simulink model "Starfighter_6DoF_runsim_waypoint"  (R2013b)
settings: Solver=ode4  StartTime=0.0  StopTime=1  FixedStep=.01  MaxStep=.004  RelTol=1e-5
values from neighbouring files (symbols this model uses):
  a = 967.78    [LocusTrans.m]    (also in runsim_Starfighter_6DoF_Waypoint.m)
  ac = [0 0 0]    [LocusTrans.m]    (also in runsim_Starfighter_6DoF_Waypoint.m)
  b = 21.9    [LocusTrans.m]    (also in runsim_Starfighter_6DoF_Waypoint.m)
  cbar = 9.6    [LocusTrans.m]    (also in runsim_Starfighter_6DoF_Waypoint.m)
  cda = 0.384    [LocusTrans.m]    (also in runsim_Starfighter_6DoF_Waypoint.m)
  cdde = 0    [LocusTrans.m]    (also in runsim_Starfighter_6DoF_Waypoint.m)
  cdo = 0.048    [LocusTrans.m]    (also in runsim_Starfighter_6DoF_Waypoint.m)
  cg = [0 0 0]    [LocusTrans.m]    (also in runsim_Starfighter_6DoF_Waypoint.m)
  cla = 2.005    [LocusTrans.m]    (also in runsim_Starfighter_6DoF_Waypoint.m)
  cladot = 0.82    [LocusTrans.m]    (also in runsim_Starfighter_6DoF_Waypoint.m)
  clb = -0.093    [LocusTrans.m]    (also in runsim_Starfighter_6DoF_Waypoint.m)
  clda = 0.0173    [LocusTrans.m]    (also in runsim_Starfighter_6DoF_Waypoint.m)
  clde = 0.523    [LocusTrans.m]    (also in runsim_Starfighter_6DoF_Waypoint.m)
  cldr = 0.0079    [LocusTrans.m]    (also in runsim_Starfighter_6DoF_Waypoint.m)
  clo = 0.122    [LocusTrans.m]    (also in runsim_Starfighter_6DoF_Waypoint.m)
  clp = -0.272    [LocusTrans.m]    (also in runsim_Starfighter_6DoF_Waypoint.m)
  clq = 1.9    [LocusTrans.m]    (also in runsim_Starfighter_6DoF_Waypoint.m)
  clr = 0.154    [LocusTrans.m]    (also in runsim_Starfighter_6DoF_Waypoint.m)
  cma = -1.308    [LocusTrans.m]    (also in runsim_Starfighter_6DoF_Waypoint.m)
  cmadot = -2.05    [LocusTrans.m]    (also in runsim_Starfighter_6DoF_Waypoint.m)
  cmde = -1.31    [LocusTrans.m]    (also in runsim_Starfighter_6DoF_Waypoint.m)
  cmo = -0.028    [LocusTrans.m]    (also in runsim_Starfighter_6DoF_Waypoint.m)
  cmq = -4.83    [LocusTrans.m]    (also in runsim_Starfighter_6DoF_Waypoint.m)
  cnb = 0.242    [LocusTrans.m]    (also in runsim_Starfighter_6DoF_Waypoint.m)
  cnda = -0.0025    [LocusTrans.m]    (also in runsim_Starfighter_6DoF_Waypoint.m)
  cndr = -0.0435    [LocusTrans.m]    (also in runsim_Starfighter_6DoF_Waypoint.m)
  cnp = -0.093    [LocusTrans.m]    (also in runsim_Starfighter_6DoF_Waypoint.m)
  cnr = -0.649    [LocusTrans.m]    (also in runsim_Starfighter_6DoF_Waypoint.m)
  cyb = -1.045    [LocusTrans.m]    (also in runsim_Starfighter_6DoF_Waypoint.m)
  cyda = 0    [LocusTrans.m]    (also in runsim_Starfighter_6DoF_Waypoint.m)
  cydr = 0.087    [LocusTrans.m]    (also in runsim_Starfighter_6DoF_Waypoint.m)
  cyp = 0    [LocusTrans.m]    (also in runsim_Starfighter_6DoF_Waypoint.m)
  cyr = 0    [LocusTrans.m]    (also in runsim_Starfighter_6DoF_Waypoint.m)
  de0 = -4.1938979*pi/180    (= -0.0731973268475)    [LocusTrans.m]    (also in runsim_Starfighter_6DoF_Waypoint.m)
  dT0 = 5795.5876705721688901230688059874    (= 5795.58767057)    [LocusTrans.m]    (also in runsim_Starfighter_6DoF_Waypoint.m = 0.4868)
  eng = [0 0 0]    [LocusTrans.m]    (also in runsim_Starfighter_6DoF_Waypoint.m)
  inialt = 55000    [runsim_Starfighter_6DoF_Waypoint.m]
  initalt = 0    [LocusTrans.m]    (also in runsim_Starfighter_6DoF_Waypoint.m = 55000)
  initeast = 0    [LocusTrans.m]    (also in runsim_Starfighter_6DoF_Waypoint.m)
  initnorth = 0    [LocusTrans.m]    (also in runsim_Starfighter_6DoF_Waypoint.m)
  initp = p0    (= 0)    [LocusTrans.m]    (also in runsim_Starfighter_6DoF_Waypoint.m)
  initpitch = theta0    (= 0.0519025210107)    [LocusTrans.m]    (also in runsim_Starfighter_6DoF_Waypoint.m)
  initq = q0    (= 0)    [LocusTrans.m]    (also in runsim_Starfighter_6DoF_Waypoint.m)
  initr = r0    (= 0)    [LocusTrans.m]    (also in runsim_Starfighter_6DoF_Waypoint.m)
  initroll = phi0    (= 0)    [LocusTrans.m]    (also in runsim_Starfighter_6DoF_Waypoint.m)
  initu = u0    [LocusTrans.m]    (also in runsim_Starfighter_6DoF_Waypoint.m)
  initv = v0    [LocusTrans.m]    (also in runsim_Starfighter_6DoF_Waypoint.m)
  initw = w0    [LocusTrans.m]    (also in runsim_Starfighter_6DoF_Waypoint.m)
  inityaw = 0.0    (= 0)    [LocusTrans.m]    (also in runsim_Starfighter_6DoF_Waypoint.m)
  Ix = 3600    [LocusTrans.m]    (also in runsim_Starfighter_6DoF_Waypoint.m)
  Ixz = 0    [LocusTrans.m]    (also in runsim_Starfighter_6DoF_Waypoint.m)
  Iy = 59000    [LocusTrans.m]    (also in runsim_Starfighter_6DoF_Waypoint.m)
  Iz = 60000    [LocusTrans.m]    (also in runsim_Starfighter_6DoF_Waypoint.m)
  K_phi = 10    [runsim_Starfighter_6DoF_Waypoint.m]
  rho = .002378*(1-.0000068756*     h)^4.2561    (= 0.000314842619782)    [LocusTrans.m]    (also in runsim_Starfighter_6DoF_Waypoint.m)
  sw = 196    [LocusTrans.m]    (also in runsim_Starfighter_6DoF_Waypoint.m)
  T_max = 11905    [runsim_Starfighter_6DoF_Waypoint.m]
  u0 = Vt0*cos(alpha0)*cos(beta0)    [LocusTrans.m]    (also in runsim_Starfighter_6DoF_Waypoint.m)
  Vt0 = 1742    [Control.m]    (also in LocusTrans.m; runsim_Starfighter_6DoF_Waypoint.m)
  weight = 16300    [runsim_Starfighter_6DoF_Waypoint.m]
  Xw = (1/u0)*Xa    [LocusTrans.m]    (also in runsim_Starfighter_6DoF_Waypoint.m = 2*[52*Vt0, 104*Vt0, 104*Vt0, 52*Vt0, 0])
libraries: simulink x6, dspswit3 x1
(part 2 of 2)

== system Starfighter_6DoF_runsim_waypoint/Aircraft_Dynamics/Aerodynamics/Aero Forces and Moments/Aerodynamic Forces ==
  CD : Inport
  CY : Inport  Port=2
  CL : Inport  Port=3
  Wind Para : Inport  Port=4
  dyn(q) : Inport  Port=5
  Body to Wind : Subsystem
  Demux : Demux  Outputs=3
  Gain : Gain  Gain=-1  SaturateOnIntegerOverflow=on  OutDataTypeStr=Inherit: Same as input  ParamDataTypeStr=Inherit: Same as input
  Gain1 : Gain  Gain=-1  SaturateOnIntegerOverflow=on  OutDataTypeStr=Inherit: Same as input  ParamDataTypeStr=Inherit: Same as input
  Gain2 : Gain  Gain=sw  SaturateOnIntegerOverflow=on  OutDataTypeStr=Inherit: Same as input  ParamDataTypeStr=Inherit: Same as input
  Math Function : Math  Operator=transpose  SaturateOnIntegerOverflow=on
  Mux : Mux  Inputs=3
  Product : Product  SaturateOnIntegerOverflow=on  OutDataTypeStr=Inherit: Same as first input
  Product1 : Product  Multiplication=Matrix(*)  SaturateOnIntegerOverflow=on  OutDataTypeStr=Inherit: Same as first input
  Terminator : Terminator
  FaeroBody : Outport
  wires:
  Gain/1 -> Mux/1
  Gain1/1 -> Mux/3
  Mux/1 -> Product/1
  Gain2/1 -> Product/2
  CD/1 -> Gain/1
  CY/1 -> Mux/2
  CL/1 -> Gain1/1
  dyn(q)/1 -> Gain2/1
  Wind Para/1 -> Demux/1
  Demux/1 -> Terminator/1
  Body to Wind/1(Smatrix) -> Math Function/1
  Math Function/1 -> Product1/1
  Product/1 -> Product1/2
  Product1/1 -> FaeroBody/1
  Demux/2 -> Body to Wind/1(Alpha)
  Demux/3 -> Body to Wind/2(Beta)

== system Starfighter_6DoF_runsim_waypoint/Aircraft_Dynamics/Aerodynamics/Aero Forces and Moments/Aerodynamic Moments ==
  dyn(q) : Inport
  Croll : Inport  Port=2
  CM : Inport  Port=3
  CN : Inport  Port=4
  Mux : Mux  Inputs=2
  Mux1 : Mux  Inputs=2
  Mux2 : Mux  Inputs=2
  Mux3 : Mux  Inputs=3
  Pitch : Fcn  Expr=u[1] * sw * cbar * u[2]
  Roll : Fcn  Expr=u[1] * sw * b * u[2]
  Yaw : Fcn  Expr=u[1] * sw * b * u[2]
  Maero : Outport
  wires:
  Mux/1 -> Roll/1
  Mux1/1 -> Pitch/1
  Mux2/1 -> Yaw/1
  Pitch/1 -> Mux3/2
  Roll/1 -> Mux3/1
  Yaw/1 -> Mux3/3
  dyn(q)/1 -> Mux/1, Mux1/1, Mux2/1
  Croll/1 -> Mux/2
  CM/1 -> Mux1/2
  CN/1 -> Mux2/2
  Mux3/1 -> Maero/1

== system Starfighter_6DoF_runsim_waypoint/Aircraft_Dynamics/Equations of motion numerical integration /Kinematic Equiations/pi Bound ==
  In : Inport
  2pi : Constant  Value=2*pi
  Math Function : Math  Operator=mod  SaturateOnIntegerOverflow=on
  Sum1 : Sum  Inputs=|+-  SaturateOnIntegerOverflow=on  InputSameDT=on  OutDataTypeStr=Inherit: Same as first input
  Sum2 : Sum  Inputs=|++  SaturateOnIntegerOverflow=on  InputSameDT=on  OutDataTypeStr=Inherit: Same as first input
  pi : Constant  Value=pi
  Out : Outport
  wires:
  Sum1/1 -> Out/1
  pi/1 -> Sum1/2, Sum2/2
  Sum2/1 -> Math Function/1
  In/1 -> Sum2/1
  2pi/1 -> Math Function/2
  Math Function/1 -> Sum1/1

== system Starfighter_6DoF_runsim_waypoint/Aircraft_Dynamics/Equations of motion numerical integration /Kinematic Equiations/pi Bound1 ==
  In : Inport
  2pi : Constant  Value=2*pi
  Math Function : Math  Operator=mod  SaturateOnIntegerOverflow=on
  Sum1 : Sum  Inputs=|+-  SaturateOnIntegerOverflow=on  InputSameDT=on  OutDataTypeStr=Inherit: Same as first input
  Sum2 : Sum  Inputs=|++  SaturateOnIntegerOverflow=on  InputSameDT=on  OutDataTypeStr=Inherit: Same as first input
  pi : Constant  Value=pi
  Out : Outport
  wires:
  Sum1/1 -> Out/1
  pi/1 -> Sum1/2, Sum2/2
  Sum2/1 -> Math Function/1
  In/1 -> Sum2/1
  2pi/1 -> Math Function/2
  Math Function/1 -> Sum1/1

== system Starfighter_6DoF_runsim_waypoint/Aircraft_Dynamics/Equations of motion numerical integration /Moment Equations/Inertia Coefs ==
  note: Jx,Jy,Jz,Jxz
  note: Inertia Coefficeents
      | Page 80 Stevens and Lewis
  Inertia : Inport
  Mux : Mux  Inputs=9
  c1 : Fcn  Expr=((u[2]-u[3])*u[3] - u[4]^2)/(u[1]*u[3]-u[4]^2)
  c2 : Fcn  Expr=((u[1]-u[2]+u[3])*u[4])/(u[1]*u[3]-u[4]^2)
  c3 : Fcn  Expr=u[3]/(u[1]*u[3]-u[4]^2)
  c4 : Fcn  Expr=u[4]/(u[1]*u[3]-u[4]^2)
  c5 : Fcn  Expr=(u[3]-u[1])/u[2]
  c6 : Fcn  Expr=u[4]/u[2]
  c7 : Fcn  Expr=1/u[2]
  c8 : Fcn  Expr=(u[1]*(u[1]-u[2])+u[4]^2)/(u[1]*u[3]-u[4]^2)
  c9 : Fcn  Expr=u[1]/(u[1]*u[3]-u[4]^2)
  Iner Coef : Outport
  wires:
  Inertia/1 -> c1/1, c2/1, c3/1, c4/1, c5/1, c6/1, c7/1, c9/1, c8/1
  c1/1 -> Mux/1
  c2/1 -> Mux/2
  c3/1 -> Mux/3
  c4/1 -> Mux/4
  c5/1 -> Mux/5
  c6/1 -> Mux/6
  c7/1 -> Mux/7
  c8/1 -> Mux/8
  c9/1 -> Mux/9
  Mux/1 -> Iner Coef/1

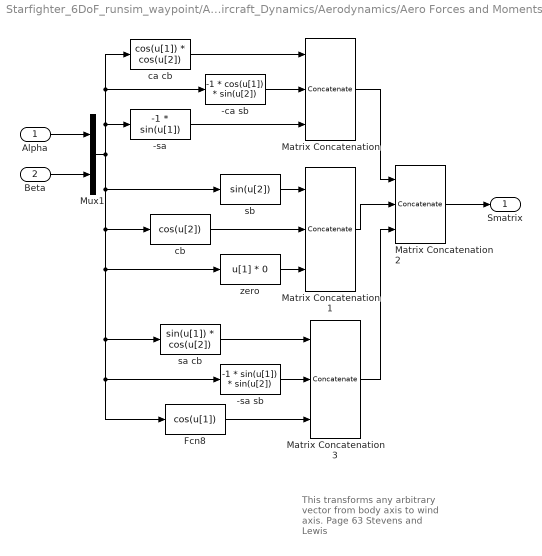
== system Starfighter_6DoF_runsim_waypoint/Aircraft_Dynamics/Aerodynamics/Aero Forces and Moments/Aerodynamic Forces/Body to Wind ==
  note: This transforms any arbitrary vector from body axis to wind axis.
      | Page 63  Stevens and Lewis
  Alpha : Inport
  Beta : Inport  Port=2
  -ca sb : Fcn  Expr=-1 * cos(u[1]) * sin(u[2])
  -sa : Fcn  Expr=-1 * sin(u[1])
  -sa sb : Fcn  Expr="-1 * sin(u[1])  * sin(u[2])"
  Fcn8 : Fcn  Expr=cos(u[1])
  Matrix Concatenation : Concatenate  NumInputs=3  Mode=Multidimensional array
  Matrix Concatenation1 : Concatenate  NumInputs=3  Mode=Multidimensional array
  Matrix Concatenation2 : Concatenate  NumInputs=3  Mode=Multidimensional array  ConcatenateDimension=2
  Matrix Concatenation3 : Concatenate  NumInputs=3  Mode=Multidimensional array
  Mux1 : Mux  Inputs=2
  ca cb : Fcn  Expr="cos(u[1]) *  cos(u[2])"
  cb : Fcn  Expr=cos(u[2])
  sa cb : Fcn  Expr=sin(u[1]) * cos(u[2])
  sb : Fcn  Expr=sin(u[2])
  zero : Fcn  Expr=u[1] * 0
  Smatrix : Outport
  wires:
  Matrix Concatenation/1 -> Matrix Concatenation2/1
  Matrix Concatenation1/1 -> Matrix Concatenation2/2
  Matrix Concatenation3/1 -> Matrix Concatenation2/3
  -ca sb/1 -> Matrix Concatenation/2
  ca cb/1 -> Matrix Concatenation/1
  -sa/1 -> Matrix Concatenation/3
  zero/1 -> Matrix Concatenation1/3
  sb/1 -> Matrix Concatenation1/1
  cb/1 -> Matrix Concatenation1/2
  sa cb/1 -> Matrix Concatenation3/1
  -sa sb/1 -> Matrix Concatenation3/2
  Fcn8/1 -> Matrix Concatenation3/3
  Mux1/1 -> ca cb/1, -ca sb/1, -sa/1, sb/1, cb/1, zero/1, sa cb/1, -sa sb/1, Fcn8/1
  Alpha/1 -> Mux1/1
  Matrix Concatenation2/1 -> Smatrix/1
  Beta/1 -> Mux1/2

== matlab function Starfighter_6DoF_runsim_waypoint/Waypoint Guidance/MATLAB Function ==
  data: d output; X input; Y input; Z input; psi_b output; count input
function [d, psi_b] = fcn(X,Y,Z,count)


Vt0 = 1742;

Xw = 2*[52*Vt0, 104*Vt0, 104*Vt0, 52*Vt0, 0];
Yw = [30*Vt0, -30*Vt0, 30*Vt0, -30*Vt0, 0];
hw = 55000;
count = round(count); 
if count<=5 && count>0
d = sqrt((X - Xw(count))^2 + (Y - Yw(count))^2);
psi_b = atan2((-Y + Yw(count)),(-X + Xw(count)));


else
    
    d = 0;
    psi_b = 0;
end
